simulink model "rectifier_2017a"  (R2017a)
settings: Solver=ode23t  StartTime=0.0  StopTime=45  FixedStep=Ts  MaxStep=Ts  RelTol=1e-4
undefined symbols (not defined in the file or in its folder): C1, Ts
libraries: powerlib x14, powerlib_meascontrol x4
settings Model: Creator=jvr2131  LastModifiedBy=jvr2131
settings DataIOCC: SaveFormat=Array
settings OptimizationCC: BlockReduction=off  BooleanDataType=off  LifeSpan=inf
settings DebuggingCC: SaveWithParameterizedLinksMsg=none  UnderspecifiedInitializationDetection=Classic  MergeDetectMultiDrivingBlocksExec=none  SignalResolutionControl=TryResolveAllWithWarning  MultiTaskDSMMsg=warning  MultiTaskCondExecSysMsg=none  StateNameClashWarn=warning  StrictBusMsg=None  SFUnexpectedBacktrackingDiag=warning  SFNoUnconditionalDefaultTransitionDiag=warning  SFExecutionAtInitializationDiag=none
settings HardwareCC: ProdBitPerPointer=32  ProdBitPerSizeT=32  ProdBitPerPtrDiffT=32  ProdLargestAtomicFloat=None  ProdIntDivRoundTo=Undefined  ProdEndianess=Unspecified  ProdWordSize=32  ProdHWDeviceType=32-bit Generic  TargetUnknown=on
settings ModelReferenceCC: PropagateSignalLabelsOutOfModel=off
settings GRTTargetCC: TargetLangStandard=C89/C90 (ANSI)  GeneratePreprocessorConditionals=Disable all
settings ConfigComp: CovMetricSettings=dw  CovHtmlReporting=on  CovSaveCumulativeToWorkspaceVar=on  CovSaveSingleToWorkspaceVar=on  CovExternalEMLEnable=off
settings SimscapeCC: SimscapeNormalizeSystem=off

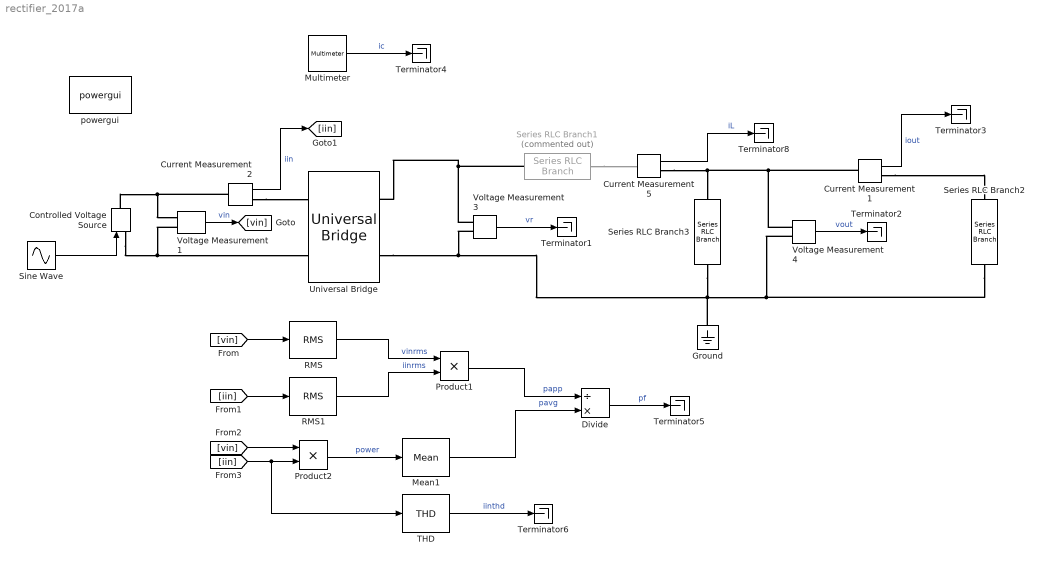
== system rectifier_2017a ==
  Controlled Voltage Source : powerlib/Electrical Sources/Controlled Voltage Source  Initialize=on  Source_Type=AC  Amplitude=0  Phase=0  Frequency=0  Measurements=None
  Current Measurement1 : powerlib/Measurements/Current Measurement  PhasorSimulation=off  OutputType=Complex  PSBequivalent=0
  Current Measurement2 : powerlib/Measurements/Current Measurement  PhasorSimulation=off  OutputType=Complex  PSBequivalent=0
  Current Measurement5 : powerlib/Measurements/Current Measurement  PhasorSimulation=off  OutputType=Complex  PSBequivalent=0
  Divide : Product  Inputs=/*
  Ground : powerlib/Elements/Ground  LConnTagsString=a
  Mean1 : powerlib_meascontrol/Measurements/Mean  Freq=50  Vinit=0  Ts=0
  Multimeter : powerlib/Measurements/Multimeter  PhasorSimulation=off  OutputType=Complex  sel=1  L=1  Gain=0  yselected={}  PSBOutputType=1  PSBequivalent=0  AxesSetting=[0,0.1,-100,100]  Display=0  SavedBlockNames=-11
  Product1 : Product
  Product2 : Product
  RMS : powerlib_meascontrol/Measurements/RMS  TrueRMS=on  Freq=50  RMSInit=120  Ts=0
  RMS1 : powerlib_meascontrol/Measurements/RMS  TrueRMS=on  Freq=50  RMSInit=120  Ts=0
  Series RLC Branch1 : powerlib/Elements/Series RLC Branch  Commented=on  LConnTagsString=__new0  RConnTagsString=__new0  BranchType=L  Resistance=1  Inductance=40.56e-3  SetiL0=off  InitialCurrent=0  Capacitance=C1  Setx0=on  InitialVoltage=Vm  Measurements=None
  Series RLC Branch2 : powerlib/Elements/Series RLC Branch  LConnTagsString=__new0  RConnTagsString=__new0  BranchType=R  Resistance=10  Inductance=1e-3  SetiL0=off  InitialCurrent=0  Capacitance=C1  Setx0=on  InitialVoltage=Vm  Measurements=None
  Series RLC Branch3 : powerlib/Elements/Series RLC Branch  LConnTagsString=__new0  RConnTagsString=__new0  BranchType=C  Resistance=1  Inductance=1e-3  SetiL0=off  InitialCurrent=0  Capacitance=100e-3  Setx0=off  InitialVoltage=Vm  Measurements=Branch current
  Sine Wave : Sin  Amplitude=230*sqrt(2)  Frequency=2*pi*50  SampleTime=0
  THD : powerlib_meascontrol/Measurements/THD  Freq=50  Ts=0
  Terminator{1..6,8} (7 alike) : Terminator
  Universal Bridge : powerlib/Power Electronics/Universal Bridge  Arms=2  SnubberResistance=1e5  SnubberCapacitance=inf  Device=Diodes  Ron=100e-3  Lon=0  ForwardVoltages="[  0  0  ]"  ForwardVoltage=0  GTOparameters=[ 10e-6 , 20e-6 ]  IGBTparameters=[ 1e-6 , 2e-6 ]  Measurements=None  Measurements_2=None  converterType=Rectifier
  Voltage Measurement1 : powerlib/Measurements/Voltage Measurement  PhasorSimulation=off  OutputType=Complex  PSBequivalent=0
  Voltage Measurement3 : powerlib/Measurements/Voltage Measurement  PhasorSimulation=off  OutputType=Complex  PSBequivalent=0
  Voltage Measurement4 : powerlib/Measurements/Voltage Measurement  PhasorSimulation=off  OutputType=Complex  PSBequivalent=0
  powergui : powerlib/powergui  Priority=1  SimulationMode=Continuous  SampleTime=Ts  frequency=60  Iterations=50  frequencyindice=0  Pbase=100e6  ErrMax=1e-4  UnitsV=kV  UnitsW=MW  buscounter=0  FunctionMessages=off  echomessages=off  EnableUseOfTLC=off  CurrentSourceSwitches=off  DisableSnubberDevices=off  DisableRonSwitches=off  DisableVfSwitches=off  DisplayEquations=off  SolverType=Tustin/Backward Euler (TBE)  Interpol=off  ExternalGateDelay=off  methode=off  Ts=100  x0status=blocks  SPID=off  SwTol=0  HookPort=off  RestoreLinks=warning  ResistiveCurrentMeasurement=off  Frange=[0:2:500]  Ylog=off  Xlog=on  ShowGrid=off  save=off  variable=ZData  structure=0  ZoomFFT=off  StartTime=0.0  cycles=1  DisplayStyle=1  fundamental=60  FreqAxis=off  MaxFrequency=1000  frequencyindicesteady=1  RmsSteady=1  display=off
  wires:
  Current Measurement2/1 -> [iin]  "iin"
  Voltage Measurement3/1 -> Terminator1/1  "vr"
  Current Measurement5/1 -> Terminator8/1  "iL"
  Voltage Measurement4/1 -> Terminator2/1  "vout"
  Current Measurement1/1 -> Terminator3/1  "iout"
  Multimeter/1 -> Terminator4/1  "ic"
  Sine Wave/1 -> Controlled Voltage Source/1
  RMS/1 -> Product1/1  "vinrms"
  RMS1/1 -> Product1/2  "iinrms"
  Voltage Measurement1/1 -> [vin]  "vin"
  [vin] -> RMS/1
  [iin] -> RMS1/1
  [iin] -> THD/1, Product2/2
  Product2/1 -> Mean1/1  "power"
  Mean1/1 -> Divide/2  "pavg"
  Product1/1 -> Divide/1  "papp"
  Divide/1 -> Terminator5/1  "pf"
  THD/1 -> Terminator6/1  "iinthd"
  [vin] -> Product2/1
  connections:
  Current Measurement2/LConn1 -- Controlled Voltage Source/RConn1 -- Voltage Measurement1/LConn1
  Voltage Measurement1/LConn2 -- Controlled Voltage Source/LConn1 -- Universal Bridge/LConn2
  Current Measurement2/RConn1 -- Universal Bridge/LConn1
  Series RLC Branch2/RConn1 -- Voltage Measurement3/LConn2 -- Universal Bridge/RConn2 -- Series RLC Branch3/RConn1 -- Ground/LConn1 -- Voltage Measurement4/LConn2
  Current Measurement5/RConn1 -- Voltage Measurement4/LConn1 -- Current Measurement1/LConn1 -- Series RLC Branch3/LConn1
  Current Measurement1/RConn1 -- Series RLC Branch2/LConn1
  Voltage Measurement3/LConn1 -- Series RLC Branch1/RConn1 -- Universal Bridge/RConn1
  Series RLC Branch1/LConn1 -- Current Measurement5/LConn1
